simulink library "find6DOFSnellMin_cl"  (R2018b)
settings: Solver=VariableStepAuto  StartTime=0.0  StopTime=10.0  RelTol=1e-3
undefined symbols (not defined in the file or in its folder): params
libraries: rayTrace_ul x4, powellsMethodMin_ul x1
settings Model: Creator=MAE-NCSUCORE  LastModifiedBy=MAE-NCSUCORE

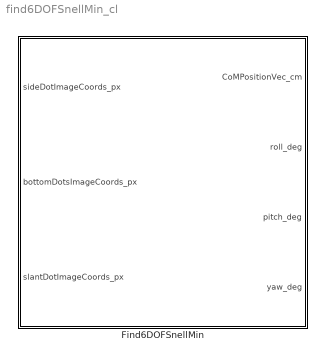
== system find6DOFSnellMin_cl ==
  Find6DOFSnellMin : Subsystem  mask{imageDims_px=params.sideImageSize_px.Value, initialCoMPositionVec_cm=params.initCoMPosVec_cm.Value, initialEulerAngles_deg=params.initEulerAng_deg.Value, indxOfRefVec=params.indexOfRefractionA.Value, glassThickness_cm=params.glassThickness_cm.Value, cameraFOVAngles_deg=params.cameraFOV_deg.Value, sideEulerAngles_deg=params.sideCamEulAng_deg.Value, sideCamPositionVec_cm=params.sideCamPosVec_cm.Value, sideCamDistToGlass_cm=params.sideDistancetoGlass_cm.Value, botEulerAngles_deg=params.botCamEulAng_deg.Value, botCamPositionVec_cm=params.botCamPosVec_cm.Value, botCamDistToGlass_cm=params.botDistancetoGlass_cm.Value, slantEulerAngles_deg=params.slntCamEulAng_deg.Value, slantCamPositionVec_cm=params.slntCamPosVec_cm.Value, slantCamDistToGlass_cm=params.slntDistancetoGlass_cm.Value, sideSeparation_cm=params.sideDotSepDist_cm.Value, sidePositionVecBF_cm=params.sideDotPosVec_cm.Value, bottomASeparation_cm=params.botADotSepDist_cm.Value, botAPositionVecBF_cm=params.botADotPosVec_cm.Value, bottomBSeparation_cm=params.botBDotSepDist_cm.Value, botBPositionVecBF_cm=params.botBDotPosVec_cm.Value}
      mask prompts: imageDims_px "Image Dimensions [rows, cols] [px]"; initialCoMPositionVec_cm "Initial CoM Position Vector [cm]"; initialEulerAngles_deg "Initial Euler Angles [deg]"; indxOfRefVec "Indices of refraction, [air glass water]"; glassThickness_cm "Glass thickness [cm]"; cameraFOVAngles_deg "Field of View Angles [horiz, vert] [deg]"; sideEulerAngles_deg "Euler Angles [roll pitch yaw] [deg]"; sideCamPositionVec_cm "Position Vector [cm]"; sideCamDistToGlass_cm "Distance to Glass [cm]"; botEulerAngles_deg "Euler Angles [roll pitch yaw]  [deg]"; botCamPositionVec_cm "Position Vector [cm]"; botCamDistToGlass_cm "Distance to Glass [cm]"; slantEulerAngles_deg "Euler Angles [roll pitch yaw]  [deg]"; slantCamPositionVec_cm "Position Vec [cm]"; slantCamDistToGlass_cm "Distance to Glass [cm]"; sideSeparation_cm "Separation Distance [cm]"; sidePositionVecBF_cm "Centroid Position in Body Frame [cm]"; bottomASeparation_cm "Separation Distance [cm]"; botAPositionVecBF_cm "Centroid Position in Body Frame [cm]"; bottomBSeparation_cm "Separation Distance [cm]"; botBPositionVecBF_cm "Centroid Position in Body Frame [cm]"
      mask init:
      | find6DOFSnellMin_init;
      mask DialogControl Container4 Prompt: Camera Properties
      mask DialogControl Container7 Prompt: Side Camera
      mask DialogControl Container8 Prompt: Bottom Camera
      mask DialogControl Container9 Prompt: Slant Camera
      mask DialogControl Container13 Prompt: Dot Properties
      mask DialogControl Container14 Prompt: Side Dots
      mask DialogControl Container15 Prompt: Bottom Dot Set A
      mask DialogControl Container16 Prompt: Bottom Dot Set B
      mask Display:
      | image('blockImage.png',[.2, .2, .6, .6],'on');
      | 
      | port_label('input',1,'Side')
      | port_label('input',2,'Bottom')
      | port_label('input',3,'Slant')
      | 
      | port_label('output',1,'CoMPosVec_cm')
      | port_label('output',2,'roll_rad')
      | port_label('output',3,'pitch_rad')
      | port_label('output',4,'yaw_rad')
      | 
      | % port_label('output',4,'err')
      | % port_label('output',5,'rxRaw')
      | % port_label('output',6,'ryRaw')
      | 
      | text(0.5, 1, 'Snells Law - Resolve 6 DOF', 'horizontalAlignment', 'center', ...
      |   'verticalAlignment', 'top')

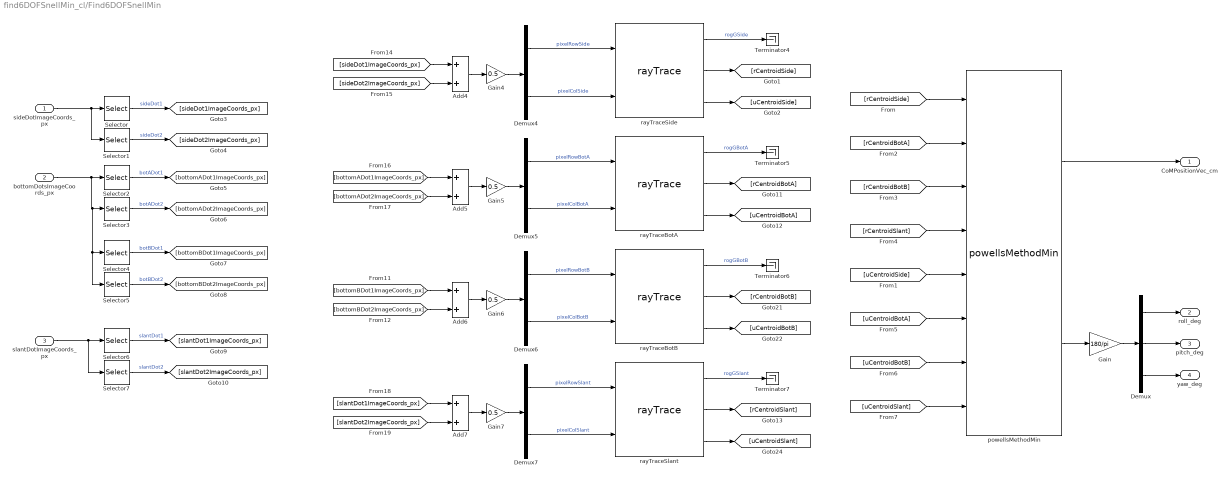
== system find6DOFSnellMin_cl/Find6DOFSnellMin ==
  sideDotImageCoords_px : Inport
  bottomDotsImageCoords_px : Inport  Port=2
  slantDotImageCoords_px : Inport  Port=3
  Add{4..7} (4 alike) : Sum
  Demux : Demux  Outputs=3
  Demux{4..7} (4 alike) : Demux  Outputs=2
  Gain : Gain  Gain=180/pi
  Gain{4..7} (4 alike) : Gain  Gain=0.5
  Selector : Selector  InputPortWidth=4  IndexOptions=Index vector (dialog)  Indices=[1 2]  OutputSizes=1
  Selector1 : Selector  InputPortWidth=4  IndexOptions=Index vector (dialog)  Indices=[3 4]  OutputSizes=1
  Selector2 : Selector  InputPortWidth=8  IndexOptions=Index vector (dialog)  Indices=[1 2]  OutputSizes=1
  Selector3 : Selector  InputPortWidth=8  IndexOptions=Index vector (dialog)  Indices=[3 4]  OutputSizes=1
  Selector4 : Selector  InputPortWidth=8  IndexOptions=Index vector (dialog)  Indices=[5 6]  OutputSizes=1
  Selector5 : Selector  InputPortWidth=8  IndexOptions=Index vector (dialog)  Indices=[7 8]  OutputSizes=1
  Selector6 : Selector  InputPortWidth=4  IndexOptions=Index vector (dialog)  Indices=[1 2]  OutputSizes=1
  Selector7 : Selector  InputPortWidth=4  IndexOptions=Index vector (dialog)  Indices=[3 4]  OutputSizes=1
  Terminator{4..7} (4 alike) : Terminator
  powellsMethodMin : powellsMethodMin_ul/powellsMethodMin  sideDotPosVec_cm=sidePositionVecBF_cm  botADotPosVec_cm=botAPositionVecBF_cm  botBDotPosVec_cm=botBPositionVecBF_cm  initialCoMPositionVec_cm=initialCoMPositionVec_cm  initialEulerAngles_rad=initialEulerAngles_rad
  rayTraceBotA : rayTrace_ul/rayTrace  camPosVec_cm=botCamPositionVec_cm  camEulAngles_deg=botEulerAngles_deg  dist2Glass_cm=botCamDistToGlass_cm  indOfRefVec=indxOfRefVec  glassPlane=1  glassThickness_cm=glassThickness_cm  imageDimsVec_px=imageDims_px  camFOV_deg=cameraFOVAngles_deg
  rayTraceBotB : rayTrace_ul/rayTrace  camPosVec_cm=botCamPositionVec_cm  camEulAngles_deg=botEulerAngles_deg  dist2Glass_cm=botCamDistToGlass_cm  indOfRefVec=indxOfRefVec  glassPlane=1  glassThickness_cm=glassThickness_cm  imageDimsVec_px=imageDims_px  camFOV_deg=cameraFOVAngles_deg
  rayTraceSide : rayTrace_ul/rayTrace  camPosVec_cm=sideCamPositionVec_cm  camEulAngles_deg=sideEulerAngles_deg  dist2Glass_cm=sideCamDistToGlass_cm  indOfRefVec=indxOfRefVec  glassPlane=2  glassThickness_cm=glassThickness_cm  imageDimsVec_px=imageDims_px  camFOV_deg=cameraFOVAngles_deg
  rayTraceSlant : rayTrace_ul/rayTrace  camPosVec_cm=slantCamPositionVec_cm  camEulAngles_deg=slantEulerAngles_deg  dist2Glass_cm=slantCamDistToGlass_cm  indOfRefVec=indxOfRefVec  glassPlane=1  glassThickness_cm=glassThickness_cm  imageDimsVec_px=imageDims_px  camFOV_deg=cameraFOVAngles_deg
  CoMPositionVec_cm : Outport
  roll_deg : Outport  Port=2
  pitch_deg : Outport  Port=3
  yaw_deg : Outport  Port=4
  wires:
  Selector6/1 -> [slantDot1ImageCoords_px]  "slantDot1"
  Gain6/1 -> Demux6/1
  Add6/1 -> Gain6/1
  rayTraceBotA/2 -> [rCentroidBotA]
  Demux5/2 -> rayTraceBotA/2  "pixelColBotA"
  [bottomADot1ImageCoords_px] -> Add5/1
  Selector4/1 -> [bottomBDot1ImageCoords_px]  "botBDot1"
  Selector/1 -> [sideDot1ImageCoords_px]  "sideDot1"
  [sideDot1ImageCoords_px] -> Add4/1
  Add7/1 -> Gain7/1
  rayTraceSlant/3 -> [uCentroidSlant]
  Add5/1 -> Gain5/1
  rayTraceSide/2 -> [rCentroidSide]
  bottomDotsImageCoords_px/1 -> Selector2/1, Selector3/1, Selector4/1, Selector5/1
  rayTraceBotB/1 -> Terminator6/1  "rogGBotB"
  rayTraceSide/1 -> Terminator4/1  "rogGSide"
  rayTraceBotA/1 -> Terminator5/1  "rogGBotA"
  Demux4/1 -> rayTraceSide/1  "pixelRowSide"
  Gain4/1 -> Demux4/1
  Gain5/1 -> Demux5/1
  Add4/1 -> Gain4/1
  Gain7/1 -> Demux7/1
  Demux6/1 -> rayTraceBotB/1  "pixelRowBotB"
  rayTraceSide/3 -> [uCentroidSide]
  rayTraceBotB/3 -> [uCentroidBotB]
  Demux7/1 -> rayTraceSlant/1  "pixelRowSlant"
  sideDotImageCoords_px/1 -> Selector/1, Selector1/1
  Demux6/2 -> rayTraceBotB/2  "pixelColBotB"
  rayTraceSlant/1 -> Terminator7/1  "rogGSlant"
  rayTraceBotA/3 -> [uCentroidBotA]
  [slantDot2ImageCoords_px] -> Add7/2
  Demux5/1 -> rayTraceBotA/1  "pixelRowBotA"
  rayTraceBotB/2 -> [rCentroidBotB]
  slantDotImageCoords_px/1 -> Selector6/1, Selector7/1
  [sideDot2ImageCoords_px] -> Add4/2
  [slantDot1ImageCoords_px] -> Add7/1
  Demux7/2 -> rayTraceSlant/2  "pixelColSlant"
  rayTraceSlant/2 -> [rCentroidSlant]
  [bottomBDot2ImageCoords_px] -> Add6/2
  [bottomADot2ImageCoords_px] -> Add5/2
  Demux4/2 -> rayTraceSide/2  "pixelColSide"
  [bottomBDot1ImageCoords_px] -> Add6/1
  Selector1/1 -> [sideDot2ImageCoords_px]  "sideDot2"
  Selector5/1 -> [bottomBDot2ImageCoords_px]  "botBDot2"
  Selector2/1 -> [bottomADot1ImageCoords_px]  "botADot1"
  Selector3/1 -> [bottomADot2ImageCoords_px]  "botADot2"
  Selector7/1 -> [slantDot2ImageCoords_px]  "slantDot2"
  [uCentroidSlant] -> powellsMethodMin/8
  [uCentroidBotB] -> powellsMethodMin/7
  powellsMethodMin/1 -> CoMPositionVec_cm/1
  powellsMethodMin/2 -> Gain/1
  Gain/1 -> Demux/1
  Demux/1 -> roll_deg/1
  Demux/3 -> yaw_deg/1
  Demux/2 -> pitch_deg/1
  [rCentroidSide] -> powellsMethodMin/1
  [rCentroidBotA] -> powellsMethodMin/2
  [uCentroidBotA] -> powellsMethodMin/6
  [uCentroidSide] -> powellsMethodMin/5
  [rCentroidSlant] -> powellsMethodMin/4
  [rCentroidBotB] -> powellsMethodMin/3
